simulink library "Coord_BodyToLeg"  (R2014b)
settings: Solver=ode45  StartTime=0.0  StopTime=10.0  RelTol=1e-3
settings Model: Creator=Sebastian  LastModifiedBy=Sebastian

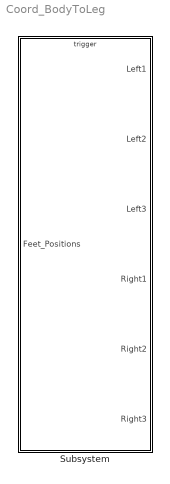
== system Coord_BodyToLeg ==
  Subsystem : Subsystem

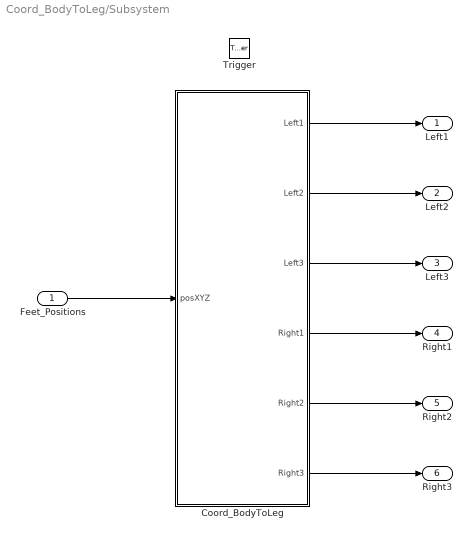
== system Coord_BodyToLeg/Subsystem ==
  Feet_Positions : Inport
  Trigger : TriggerPort  PortDimensions=1
  Coord_BodyToLeg : MATLAB Function  TreatAsAtomicUnit=on
  Left1 : Outport
  Left2 : Outport  Port=2
  Left3 : Outport  Port=3
  Right1 : Outport  Port=4
  Right2 : Outport  Port=5
  Right3 : Outport  Port=6
  wires:
  Feet_Positions/1 -> Coord_BodyToLeg/1(posXYZ)
  Coord_BodyToLeg/3(Left3) -> Left3/1
  Coord_BodyToLeg/2(Left2) -> Left2/1
  Coord_BodyToLeg/6(Right3) -> Right3/1
  Coord_BodyToLeg/4(Right1) -> Right1/1
  Coord_BodyToLeg/1(Left1) -> Left1/1
  Coord_BodyToLeg/5(Right2) -> Right2/1

== matlab function Coord_BodyToLeg/Subsystem/Coord_BodyToLeg ==
  data: Left1 output; Left2 output; Left3 output; Right1 output; Right2 output; Right3 output; posXYZ input
function [Left1,Left2,Left3,Right1,Right2,Right3] = fcn(posXYZ)

%Syntax
%x1 ... x6
%y1 ... y6
%z1 ... z6

posXYZ=posXYZ';%x y z
out=zeros(3,6);
posXY=posXYZ(1:2,:);

%Offset measured from the origin of the main body
%Ordning L1 L2 L3 R1 R2 R3
offset=zeros(2,6);
offset(1,:)=[-60.91 -103.5 -60.91 60.91 103.5 60.91];%x offset
offset(2,:)=[121.91 0 -121.91 121.91 0 -121.91];%y offset

% Rotation Z based on origo on main body
angels= [45 90 135 -45 -90 -135];


for i=1:6
    ang=angels(i);
    R2=[cosd(ang) sind(ang) ;
        -sind(ang) cosd(ang)];
    
    R=[-cosd(ang) -sind(ang) ;
        sind(ang) -cosd(ang)];
    
    %Translation of origo
    R=R*offset(:,i);
    
    posXY(:,i)=[R2 R]*[posXY(:,i); 1];
    
end

%Create the output vector
out(1:2,:)=posXY;
out(3,:)=posXYZ(3,:);

Left1=round(out(:,1));
Left2=round(out(:,2));
Left3=round(out(:,3));
Right1=round(out(:,4));
Right2=round(out(:,5));
Right3=round(out(:,6));
